simulink model "FMU_Seperator"  (R2020b)
settings: Solver=FixedStepAuto  StartTime=0.0  StopTime=Inf  FixedStep=ts  RelTol=1e-3
model workspace (MAT data in the model file):
  ts = 0.01
settings Model: Creator=kaebi  LastModifiedBy=kaebi
settings OptimizationCC: DefaultParameterBehavior=Inlined  LocalBlockOutputs=off
settings RTWCC: GenCodeOnly=on

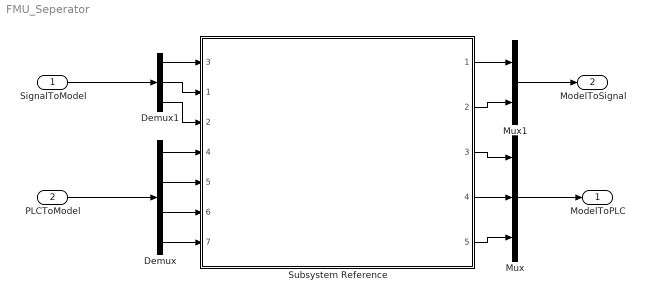
== system FMU_Seperator ==
  SignalToModel : Inport
  PLCToModel : Inport  Port=2
  Demux : Demux
  Demux1 : Demux  Outputs=3
  Mux : Mux  Inputs=3
  Mux1 : Mux  Inputs=2
  Subsystem Reference : Subsystem  ReferencedSubsystem=SubSystemVereinzelung
      settings: PortSchema="{\"entries\":[{\"content\":{\"sides\":[{\"content\":{\"connectorIds\":[\"In3\",\"In1\",\"In2\",\"In4\",\"In5\",\"In6\",\"In7\"]},\"type\":\"ConnectorPlacement.EquallySpacedRectSide\",\"uuid\":\"daf4ed04-6424-45fc-a5e8-18cb4a980d1b\"},{\"content\":{\"connectorIds\":[\"Out1\",\"Out2\",\"Out3\",\"Out4\",\"Out5\"],\"side\":\"RIGHT\"},\"type\":\"ConnectorPlacement.EquallySpacedRectSide\",\"uuid\":\"a47e6a4e-7b46-4a71-a64b-9e4e1f0754a9\"},{\"content\":{\"connectorIds\":[],\"side\":\"TOP\"},\"type\":\"ConnectorPlacement.EquallySpacedRectSide\",\"uuid\":\"b6e6389d-18ca-4ef7-b2f9-2efea5ea42cc\"},{\"content\":{\"connectorIds\":[],\"side\":\"HIDDEN\"},\"type\":\"ConnectorPlacement.EquallySpacedRectSide\",\"uuid\":\"10fc5be0-6c45-4fde-bdc8-b0820f32b2c7\"}]},\"type\":\"ConnectorPlacement.EquallySpacedConnector\",\"uuid\":\"853d100e-9740-4092-b5d4-0ad803ea10a9\"}],\"packageUris\":[\"http://schema.mathworks.com/mf0/Connector/R2020b\"],\"version\":\"1.0\"}"
  ModelToPLC : Outport
  ModelToSignal : Outport  Port=2  OutDataTypeStr=Bus: ModelToSignal
  wires:
  Demux/1 -> Subsystem Reference/4
  Demux/2 -> Subsystem Reference/5
  Demux/3 -> Subsystem Reference/6
  Demux/4 -> Subsystem Reference/7
  PLCToModel/1 -> Demux/1
  SignalToModel/1 -> Demux1/1
  Subsystem Reference/5 -> Mux/3
  Subsystem Reference/4 -> Mux/2
  Subsystem Reference/3 -> Mux/1
  Mux/1 -> ModelToPLC/1
  Subsystem Reference/2 -> Mux1/2
  Subsystem Reference/1 -> Mux1/1
  Mux1/1 -> ModelToSignal/1
  Demux1/1 -> Subsystem Reference/3
  Demux1/2 -> Subsystem Reference/1
  Demux1/3 -> Subsystem Reference/2
